simulink model "IntMatlabFcn_sim"  (R2016b)
settings: Solver=VariableStepAuto  StartTime=0.0  StopTime=2*pi  RelTol=1e-3
values from neighbouring files (symbols this model uses):
  F = Function('F',{x},{x^2},{'x'},{'r'})    [main_IntMatlabFcn.m]
  Fode = Function('ode',{x,u},{ode},char('x','u'),char('ode'))    [main_IntMatlabFcn.m]
  G = Function('G',{x,y},{y*x^2},{'x','y'},{'r'})    [main_IntMatlabFcn.m]
  x0 = [-1;0.5]    [main_IntMatlabFcn.m]
undefined symbols (not defined in the file or in its folder): full
settings Model: Creator=Gianni  LastModifiedBy=Gianni

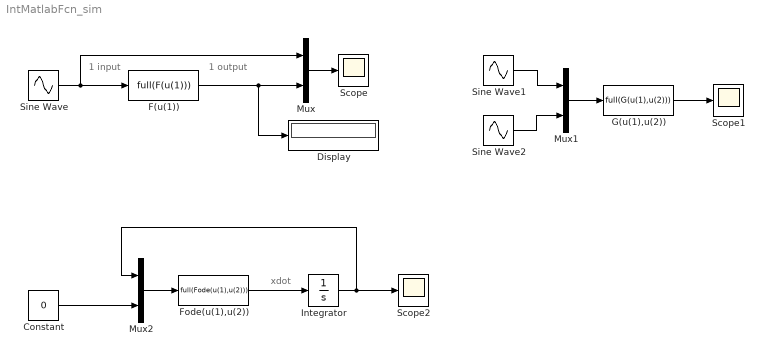
== system IntMatlabFcn_sim ==
  note: xdot
  note: 1 output
  note: 1 input
  Constant : Constant  Value=0
  Display : Display
  F(u(1)) : MATLABFcn  MATLABFcn=full(F(u(1)))
  Fode(u(1),u(2)) : MATLABFcn  MATLABFcn=full(Fode(u(1),u(2)))
  G(u(1),u(2)) : MATLABFcn  MATLABFcn=full(G(u(1),u(2)))
  Integrator : Integrator  InitialCondition=x0
  Mux : Mux  Inputs=2
  Mux1 : Mux  Inputs=2
  Mux2 : Mux  Inputs=2
  Scope : Scope
  Scope1 : Scope
  Scope2 : Scope
  Sine Wave : Sin  SampleTime=0
  Sine Wave1 : Sin  SampleTime=0
  Sine Wave2 : Sin  SampleTime=0
  wires:
  Sine Wave/1 -> F(u(1))/1, Mux/1
  Mux/1 -> Scope/1
  F(u(1))/1 -> Mux/2, Display/1
  Sine Wave1/1 -> Mux1/1
  Sine Wave2/1 -> Mux1/2
  Mux1/1 -> G(u(1),u(2))/1
  G(u(1),u(2))/1 -> Scope1/1
  Fode(u(1),u(2))/1 -> Integrator/1
  Mux2/1 -> Fode(u(1),u(2))/1
  Integrator/1 -> Scope2/1, Mux2/1
  Constant/1 -> Mux2/2
